simulink model "SupportedCoreModelElements"  (Simulink 7.8)
settings: Solver=ode45  StartTime=0.0  StopTime=10.0  RelTol=1e-3
settings Model: Creator=Arne Haber  LastModifiedBy=Arne Haber

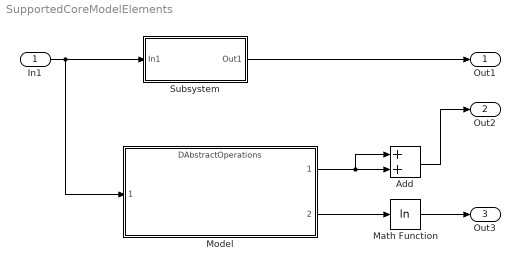
== system SupportedCoreModelElements ==
  In1 : Inport
  Add : Sum
  Math Function : Math  Operator=log  SaturateOnIntegerOverflow=on
  Model : ModelReference  ModelNameDialog=DAbstractOperations  SimulationMode=Normal  ModelReferenceVersion=1.8  CopyOfModelName=DAbstractOperations  DefaultDataLogging=on
  Subsystem : Subsystem
  Out1 : Outport
  Out2 : Outport  Port=2
  Out3 : Outport  Port=3
  wires:
  In1/1 -> Subsystem/1(In1), Model/1
  Subsystem/1(Out1) -> Out1/1
  Model/1 -> Add/1, Add/2
  Add/1 -> Out2/1
  Model/2 -> Math Function/1
  Math Function/1 -> Out3/1

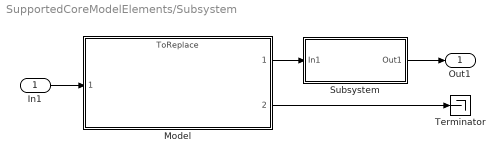
== system SupportedCoreModelElements/Subsystem ==
  In1 : Inport
  Model : ModelReference  ModelNameDialog=ToReplace  SimulationMode=Normal  ModelReferenceVersion=1.1  CopyOfModelName=ToReplace  DefaultDataLogging=on
  Subsystem : Subsystem
  Terminator : Terminator
  Out1 : Outport
  wires:
  In1/1 -> Model/1
  Subsystem/1(Out1) -> Out1/1
  Model/1 -> Subsystem/1(In1)
  Model/2 -> Terminator/1

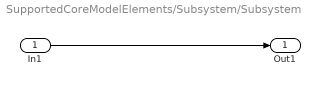
== system SupportedCoreModelElements/Subsystem/Subsystem ==
  In1 : Inport
  Out1 : Outport
  wires:
  In1/1 -> Out1/1
